simulink model "k1visbs"  (Simulink 8.5)
settings: Solver=ode45  StartTime=0.0  StopTime=10.0  RelTol=1e-3
undefined symbols (not defined in the file): AC, FOUROSEM_OPLEV_DAMP_MASTER, SIXOSEM_F_STAGE_MASTER, SIXOSEM_F_WD_AC_MASTER
libraries: cdsEpicsOut x82, cdsFilt x57, cdsTP x36, cdsFiltCtrl x16, VIS_LIB x14, cdsMuxMatrix x13, cdsEpicsIn x10, cdsEpicsBinIn x6, cdsRms x6, STATE_BIO_MASTER x4, lockin x4, cdsFunctionCall x4
(part 2 of 8)

== system k1visbs/BS/TEST ==
  In1 : Inport
  In4 : Inport  Port=2
  In7 : Inport  Port=3
  In10 : Inport  Port=4
  CH1 : cdsFiltCtrl/IIR FM with control  Tag=cdsFiltCtrl  Description=|
      | cdsFiltCntrl is the standard IIR filter module (exactly the same as cdsFilt) but with added control data output 'Ctrl'. Filter module digital signal output appears on the first output, which is called 'Val'. 'Ctrl' output has a bit pattern encoding the state of filter's on/off switches (FM1 through FM10). The bit values are:
      |                                                                                                                                                                                                                                                                                                                                       
      | module 	hex	dec                                                                                                                                                                                                                                                                                                                       
      | -----------------------                                                                                                                                                                                                                                                                                                               
      | FM1	0x20                    32                                                                                                                                                                                                                                                                                                        
      | FM2	0x80                     128                                                                                                                                                                                                                                                                                                      
      | FM3	0x200                   512                                                                                                                                                                                                                                                                                                       
      | FM4	0x800                   2048                                                                                                                                                                                                                                                                                                      
      | FM5	0x2000                 8192                                                                                                                                                                                                                                                                                                       
      | FM6	0x8000                 32768                                                                                                                                                                                                                                                                                                      
      | FM7	0x20000                131072                                                                                                                                                                                                                                                                                                     
      | FM8	0x80000                 524288                                                                                                                                                                                                                                                                                                    
      | FM9	0x200000               2097152                                                                                                                                                                                                                                                                                                    
      | FM10	0x800000               8388608                                                                                                                                                                                                                                                                                                   
      |                                                                                                                                                                                                                                                                                                                                       
      | This bit data can be used to drive some other switches or it can be output using a binary I/O module.
      settings: AttributesFormatString=%<Tag>
  CH2 : cdsFiltCtrl/IIR FM with control  Tag=cdsFiltCtrl  Description=|
      | cdsFiltCntrl is the standard IIR filter module (exactly the same as cdsFilt) but with added control data output 'Ctrl'. Filter module digital signal output appears on the first output, which is called 'Val'. 'Ctrl' output has a bit pattern encoding the state of filter's on/off switches (FM1 through FM10). The bit values are:
      |                                                                                                                                                                                                                                                                                                                                       
      | module 	hex	dec                                                                                                                                                                                                                                                                                                                       
      | -----------------------                                                                                                                                                                                                                                                                                                               
      | FM1	0x20                    32                                                                                                                                                                                                                                                                                                        
      | FM2	0x80                     128                                                                                                                                                                                                                                                                                                      
      | FM3	0x200                   512                                                                                                                                                                                                                                                                                                       
      | FM4	0x800                   2048                                                                                                                                                                                                                                                                                                      
      | FM5	0x2000                 8192                                                                                                                                                                                                                                                                                                       
      | FM6	0x8000                 32768                                                                                                                                                                                                                                                                                                      
      | FM7	0x20000                131072                                                                                                                                                                                                                                                                                                     
      | FM8	0x80000                 524288                                                                                                                                                                                                                                                                                                    
      | FM9	0x200000               2097152                                                                                                                                                                                                                                                                                                    
      | FM10	0x800000               8388608                                                                                                                                                                                                                                                                                                   
      |                                                                                                                                                                                                                                                                                                                                       
      | This bit data can be used to drive some other switches or it can be output using a binary I/O module.
      settings: AttributesFormatString=%<Tag>
  CH3 : cdsFiltCtrl/IIR FM with control  Tag=cdsFiltCtrl  Description=|
      | cdsFiltCntrl is the standard IIR filter module (exactly the same as cdsFilt) but with added control data output 'Ctrl'. Filter module digital signal output appears on the first output, which is called 'Val'. 'Ctrl' output has a bit pattern encoding the state of filter's on/off switches (FM1 through FM10). The bit values are:
      |                                                                                                                                                                                                                                                                                                                                       
      | module 	hex	dec                                                                                                                                                                                                                                                                                                                       
      | -----------------------                                                                                                                                                                                                                                                                                                               
      | FM1	0x20                    32                                                                                                                                                                                                                                                                                                        
      | FM2	0x80                     128                                                                                                                                                                                                                                                                                                      
      | FM3	0x200                   512                                                                                                                                                                                                                                                                                                       
      | FM4	0x800                   2048                                                                                                                                                                                                                                                                                                      
      | FM5	0x2000                 8192                                                                                                                                                                                                                                                                                                       
      | FM6	0x8000                 32768                                                                                                                                                                                                                                                                                                      
      | FM7	0x20000                131072                                                                                                                                                                                                                                                                                                     
      | FM8	0x80000                 524288                                                                                                                                                                                                                                                                                                    
      | FM9	0x200000               2097152                                                                                                                                                                                                                                                                                                    
      | FM10	0x800000               8388608                                                                                                                                                                                                                                                                                                   
      |                                                                                                                                                                                                                                                                                                                                       
      | This bit data can be used to drive some other switches or it can be output using a binary I/O module.
      settings: AttributesFormatString=%<Tag>
  CH4 : cdsFiltCtrl/IIR FM with control  Tag=cdsFiltCtrl  Description=|
      | cdsFiltCntrl is the standard IIR filter module (exactly the same as cdsFilt) but with added control data output 'Ctrl'. Filter module digital signal output appears on the first output, which is called 'Val'. 'Ctrl' output has a bit pattern encoding the state of filter's on/off switches (FM1 through FM10). The bit values are:
      |                                                                                                                                                                                                                                                                                                                                       
      | module 	hex	dec                                                                                                                                                                                                                                                                                                                       
      | -----------------------                                                                                                                                                                                                                                                                                                               
      | FM1	0x20                    32                                                                                                                                                                                                                                                                                                        
      | FM2	0x80                     128                                                                                                                                                                                                                                                                                                      
      | FM3	0x200                   512                                                                                                                                                                                                                                                                                                       
      | FM4	0x800                   2048                                                                                                                                                                                                                                                                                                      
      | FM5	0x2000                 8192                                                                                                                                                                                                                                                                                                       
      | FM6	0x8000                 32768                                                                                                                                                                                                                                                                                                      
      | FM7	0x20000                131072                                                                                                                                                                                                                                                                                                     
      | FM8	0x80000                 524288                                                                                                                                                                                                                                                                                                    
      | FM9	0x200000               2097152                                                                                                                                                                                                                                                                                                    
      | FM10	0x800000               8388608                                                                                                                                                                                                                                                                                                   
      |                                                                                                                                                                                                                                                                                                                                       
      | This bit data can be used to drive some other switches or it can be output using a binary I/O module.
      settings: AttributesFormatString=%<Tag>
  Ground{1..6,19,22} (8 alike) : Ground
  Terminator{1..5,16..18} (8 alike) : Terminator
  wires:
  CH4/2 -> Terminator1/1
  Ground5/1 -> CH4/3
  Ground6/1 -> CH4/2
  Ground3/1 -> CH3/3
  Ground4/1 -> CH3/2
  Ground1/1 -> CH2/3
  Ground2/1 -> CH2/2
  CH3/2 -> Terminator18/1
  CH2/2 -> Terminator17/1
  CH1/2 -> Terminator16/1
  Ground19/1 -> CH1/3
  Ground22/1 -> CH1/2
  In10/1 -> CH4/1
  In7/1 -> CH3/1
  In1/1 -> CH1/1
  CH2/1 -> Terminator4/1
  In4/1 -> CH2/1
  CH4/1 -> Terminator2/1
  CH3/1 -> Terminator3/1
  CH1/1 -> Terminator5/1

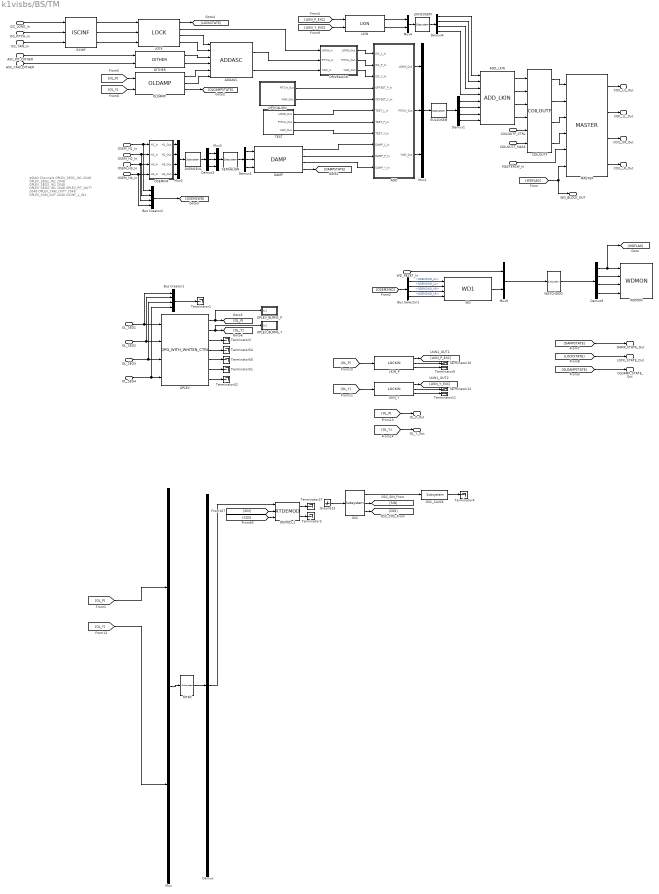
== system k1visbs/BS/TM ==
  note: #DAQ Channels
      | OPLEV_SEG1_IN1 2048
      | OPLEV_SEG2_IN1 2048
      | OPLEV_SEG3_IN1 2048
      | OPLEV_SEG4_IN1 2048
      | OPLEV_PIT_OUT* 2048
      | OPLEV_YAW_OUT* 2048
      | OPLEV_SUM_OUT 2048
      | ISCINF_L_IN1 2048
  OSEM_H1_In : Inport
  OSEM_H2_In : Inport  Port=2
  OSEM_H3_In : Inport  Port=3
  OSEM_H4_In : Inport  Port=4
  ISC_LONG_In : Inport  Port=5
  ISC_PITCH_In : Inport  Port=6
  ISC_YAW_In : Inport  Port=7
  COILOUTF_CTRL : Inport  Port=8
  COILOUTF_MASK : Inport  Port=9
  OL_SEG1 : Inport  Port=10
  OL_SEG2 : Inport  Port=11
  OL_SEG3 : Inport  Port=12
  OL_SEG4 : Inport  Port=13
  MASTERSW_In : Inport  Port=14
  WD_RESET_In : Inport  Port=15
  ASC_PIT_DITHER : Inport  Port=16
  ASC_YAW_DITHER : Inport  Port=17
  ADD : Subsystem
  ADDASC : VIS_LIB/ADDASC
  ADD_LKIN : VIS_LIB/ADD_LKIN
  Bus Creator1 : BusCreator  Inputs='OSEM2WD_UL','OSEM2WD_LL','OSEM2WD_UR','OSEM2WD_LR'
  Bus Creator2 : BusCreator  Inputs='OSEM2WD_UL','OSEM2WD_LL','OSEM2WD_UR','OSEM2WD_LR'
  Bus Selector1 : BusSelector  OutputSignals=OSEM2WD_UL,OSEM2WD_LL,OSEM2WD_UR,OSEM2WD_LR
  COILOUTF : FOUROSEM_COILOUTF_MASTER/COILOUTF
  DAMP : VIS_LIB/DAMP
  DEMOD_1 : rtdemod/RTDEMOD  Tag=top_names
  DITHER : VIS_LIB/DITHER
  DRIVEALIGN : Subsystem
  Demux : Demux  Outputs=1
  Demux1 : Demux
  Demux2 : Demux  Outputs=3
  Demux3 : Demux  Outputs=3
  Demux4 : Demux
  Demux9 : Demux
  EUL2OSEM : cdsMuxMatrix/Subsystem  Tag=cdsMuxMatrix  Description=Any size matrix. Inputs and outputs must be connected using Mux and Demux parts.
      settings: AttributesFormatString=%<Tag>
  Ground23 : Ground
  ISCINF : VIS_LIB/ISCINF
  LKIN : VIS_LIB/LKIN
  LKIN2OSEM : cdsMuxMatrix/Subsystem  Tag=cdsMuxMatrix  Description=Any size matrix. Inputs and outputs must be connected using Mux and Demux parts.
      settings: AttributesFormatString=%<Tag>
  LKIN_P : lockin/LOCKIN  Description=ADL=LOCKIN.adl
      settings: AttributesFormatString=%<Tag>
  LKIN_Y : lockin/LOCKIN  Description=ADL=LOCKIN.adl
      settings: AttributesFormatString=%<Tag>
  LOCK : VIS_LIB/LOCK
  MASTER : VIS_LIB/MASTER
  MTRX : cdsMuxMatrix/Subsystem  Tag=cdsMuxMatrix  Description=Any size matrix. Inputs and outputs must be connected using Mux and Demux parts.
      settings: AttributesFormatString=%<Tag>
  Mux : Mux  Inputs=2
  Mux1 : Mux  Inputs=3
  Mux2 : Mux
  Mux3 : Mux  Inputs=3
  Mux4 : Mux  Inputs=2
  Mux9 : Mux  Inputs=2
  OLDAMP : VIS_LIB/OLDAMP
  OPLEV : QPD/QPD_WITH_WHITEN_CTRL
  OPLEV_BLRMS_P : Subsystem
  OPLEV_BLRMS_Y : Subsystem
  OPTICALIGN : Subsystem
  OSC : cdsOsc/Subsystem  Tag=cdsOsc  Description=Oscillator
      settings: AttributesFormatString=%<Tag>
  OSC_CLOCK : cdsEpicsOut/Subsystem  Tag=cdsEpicsOutput  Description=|
      | Purpose:                                          
      | Output a FE signal to an EPICS channel.           
      |                                                   
      | Operation:                                        
      | Takes input value and passes it to EPICS record.  
      |                                                   
      | Usage:                                            
      | Name the part with the desired EPICS rrecord name.
      settings: AttributesFormatString=%<Tag>
  OSEM2EUL : cdsMuxMatrix/Subsystem  Tag=cdsMuxMatrix  Description=Any size matrix. Inputs and outputs must be connected using Mux and Demux parts.
      settings: AttributesFormatString=%<Tag>
  OSEMINF : Subsystem
  SENSALIGN : cdsMuxMatrix/Subsystem  Tag=cdsMuxMatrix  Description=Any size matrix. Inputs and outputs must be connected using Mux and Demux parts.
      settings: AttributesFormatString=%<Tag>
  TEST : Subsystem
  Terminator{1..4,9..12,27,50..52,54} (13 alike) : Terminator
  WATCHDOG : cdsFunctionCall/Subsystem  Tag=cdsFunctionCall  Description=inline OSEMWATCHDOG /opt/rtcds/userapps/release/vis/common/src/WATCHDOG.c
      settings: AttributesFormatString=%<Tag>\n%<Description>
  WD : VIS_LIB/WD1
  WDMON : VIS_LIB/WDMON
  COIL_UL_Out : Outport
  COIL_LL_Out : Outport  Port=2
  COIL_UR_Out : Outport  Port=3
  COIL_LR_Out : Outport  Port=4
  WD_BLOCK_OUT : Outport  Port=5
  DAMP_STATE_Out : Outport  Port=6
  LOCK_STATE_Out : Outport  Port=7
  OLDAMP_STATE_Out : Outport  Port=8
  OL_P_Out : Outport  Port=9
  OL_Y_Out : Outport  Port=10
  wires:
  [OL_Y] -> OL_Y_Out/1
  [OL_P] -> OL_P_Out/1
  [OL_Y] -> Mux/2
  [OL_P] -> Mux/1
  OSC/3 -> [COS]
  OSC/2 -> [SIN]
  OSC_CLOCK/1 -> Terminator4/1
  OSC/1 -> OSC_CLOCK/1
  Ground23/1 -> OSC/1
  DEMOD_1/2 -> Terminator3/1
  DEMOD_1/1 -> Terminator27/1
  [COS] -> DEMOD_1/3
  [SIN] -> DEMOD_1/2
  Demux/1 -> DEMOD_1/1
  MTRX/1 -> Demux/1
  Mux/1 -> MTRX/1
  ISCINF/3 -> LOCK/3
  ISCINF/2 -> LOCK/2
  ISCINF/1 -> LOCK/1
  ISC_PITCH_In/1 -> ISCINF/2
  ISC_LONG_In/1 -> ISCINF/1
  ISC_YAW_In/1 -> ISCINF/3
  WD/1 -> Mux9/2
  [LKIN_Y_EXC] -> LKIN/2
  [LKIN_P_EXC] -> LKIN/1
  LKIN_Y/3 -> Terminator11/1
  LKIN_Y/2 -> Terminator12/1
  [OL_Y] -> LKIN_Y/1
  LKIN_Y/1 -> [LKIN_Y_EXC]
  LKIN_P/1 -> [LKIN_P_EXC]
  LKIN_P/3 -> Terminator9/1
  LKIN_P/2 -> Terminator10/1
  [OL_P] -> LKIN_P/1
  DAMP/3 -> ADD/11(DAMP_Y_In)
  DAMP/2 -> ADD/10(DAMP_P_In)
  DAMP/1 -> ADD/9(DAMP_L_In)
  LOCK/1 -> [LOCKSTATE]
  DAMP/4 -> [DAMPSTATE]
  [OLDAMPSTATE] -> OLDAMP_STATE_Out/1
  [LOCKSTATE] -> LOCK_STATE_Out/1
  [DAMPSTATE] -> DAMP_STATE_Out/1
  MASTERSW_In/1 -> MASTER/5
  ADD_LKIN/4 -> COILOUTF/4
  ADD_LKIN/3 -> COILOUTF/3
  ADD_LKIN/2 -> COILOUTF/2
  ADD_LKIN/1 -> COILOUTF/1
  Demux1/4 -> ADD_LKIN/8
  Demux1/3 -> ADD_LKIN/7
  Demux1/2 -> ADD_LKIN/6
  Demux1/1 -> ADD_LKIN/5
  Demux4/4 -> ADD_LKIN/4
  Demux4/3 -> ADD_LKIN/3
  Demux4/2 -> ADD_LKIN/2
  LKIN/2 -> Mux4/2
  LKIN/1 -> Mux4/1
  Demux4/1 -> ADD_LKIN/1
  LKIN2OSEM/1 -> Demux4/1
  Mux4/1 -> LKIN2OSEM/1
  MASTER/4 -> COIL_LR_Out/1
  MASTER/3 -> COIL_UR_Out/1
  MASTER/2 -> COIL_LL_Out/1
  MASTER/1 -> COIL_UL_Out/1
  OPLEV/7 -> Terminator52/1
  OPLEV/6 -> Terminator51/1
  OPLEV/5 -> Terminator50/1
  OPLEV/4 -> Terminator54/1
  OLDAMP/3 -> [OLDAMPSTATE]
  OPLEV/3 -> Terminator2/1
  OPLEV/1 -> [OL_P], OPLEV_BLRMS_P/1(In1)
  OPLEV/2 -> [OL_Y], OPLEV_BLRMS_Y/1(In1)
  DRIVEALIGN/3(YAW_Out) -> ADD/3(ISC_Y_In)
  DRIVEALIGN/2(PITCH_Out) -> ADD/2(ISC_P_In)
  DRIVEALIGN/1(LONG_Out) -> ADD/1(ISC_L_In)
  ADDASC/2 -> DRIVEALIGN/3(YAW_In)
  ADDASC/1 -> DRIVEALIGN/2(PITCH_In)
  LOCK/2 -> DRIVEALIGN/1(LONG_In)
  ADD/1(LONG_Out) -> Mux1/1
  ADD/2(PITCH_Out) -> Mux1/2
  ADD/3(YAW_Out) -> Mux1/3
  OLDAMP/2 -> ADDASC/6
  OLDAMP/1 -> ADDASC/5
  DITHER/2 -> ADDASC/4
  DITHER/1 -> ADDASC/3
  LOCK/4 -> ADDASC/2
  [OL_Y] -> OLDAMP/2
  [OL_P] -> OLDAMP/1
  ASC_YAW_DITHER/1 -> DITHER/2
  ASC_PIT_DITHER/1 -> DITHER/1
  OL_SEG4/1 -> OPLEV/4, Bus Creator1/4
  OL_SEG3/1 -> Bus Creator1/3, OPLEV/3
  OL_SEG2/1 -> Bus Creator1/2, OPLEV/2
  OL_SEG1/1 -> OPLEV/1, Bus Creator1/1
  Bus Selector1/4 -> WD/4  "<OSEM2WD_LR>"
  Bus Selector1/3 -> WD/3  "<OSEM2WD_UR>"
  Bus Selector1/2 -> WD/2  "<OSEM2WD_LL>"
  Bus Selector1/1 -> WD/1  "<OSEM2WD_UL>"
  [OSEM2WD] -> Bus Selector1/1
  Demux2/3 -> DAMP/3
  Demux2/2 -> DAMP/2
  Demux2/1 -> DAMP/1
  OSEMINF/4(H4_Out) -> Mux2/4
  OSEMINF/3(H3_Out) -> Mux2/3
  OSEMINF/2(H2_Out) -> Mux2/2
  OSEMINF/1(H1_Out) -> Mux2/1
  OSEM_H4_In/1 -> Bus Creator2/4, OSEMINF/4(H4_In)
  OSEM_H3_In/1 -> Bus Creator2/3, OSEMINF/3(H3_In)
  OSEM_H2_In/1 -> Bus Creator2/2, OSEMINF/2(H2_In)
  OSEM_H1_In/1 -> Bus Creator2/1, OSEMINF/1(H1_In)
  Mux2/1 -> OSEM2EUL/1
  OSEM2EUL/1 -> Demux3/1
  Mux3/1 -> SENSALIGN/1
  SENSALIGN/1 -> Demux2/1
  Mux1/1 -> EUL2OSEM/1
  EUL2OSEM/1 -> Demux1/1
  Demux3/1 -> Mux3/1
  Demux3/2 -> Mux3/2
  Demux3/3 -> Mux3/3
  Demux9/1 -> [WDFLAG], WDMON/1
  Demux9/2 -> WDMON/2
  Demux9/3 -> WDMON/3
  Demux9/4 -> WDMON/4
  WATCHDOG/1 -> Demux9/1
  Mux9/1 -> WATCHDOG/1
  [WDFLAG] -> WD_BLOCK_OUT/1, MASTER/6
  COILOUTF/1 -> MASTER/1
  COILOUTF/2 -> MASTER/2
  COILOUTF/3 -> MASTER/3
  COILOUTF/4 -> MASTER/4
  WD_RESET_In/1 -> Mux9/1
  COILOUTF_MASK/1 -> COILOUTF/6
  COILOUTF_CTRL/1 -> COILOUTF/5
  TEST/1(LONG_Out) -> ADD/6(TEST_L_In)
  TEST/2(PITCH_Out) -> ADD/7(TEST_P_In)
  TEST/3(YAW_Out) -> ADD/8(TEST_Y_In)
  LOCK/3 -> ADDASC/1
  OPTICALIGN/1(PITCH_Out) -> ADD/4(OFFSET_P_In)
  OPTICALIGN/2(YAW_Out) -> ADD/5(OFFSET_Y_In)
  Bus Creator2/1 -> [OSEM2WD]
  Bus Creator1/1 -> Terminator1/1

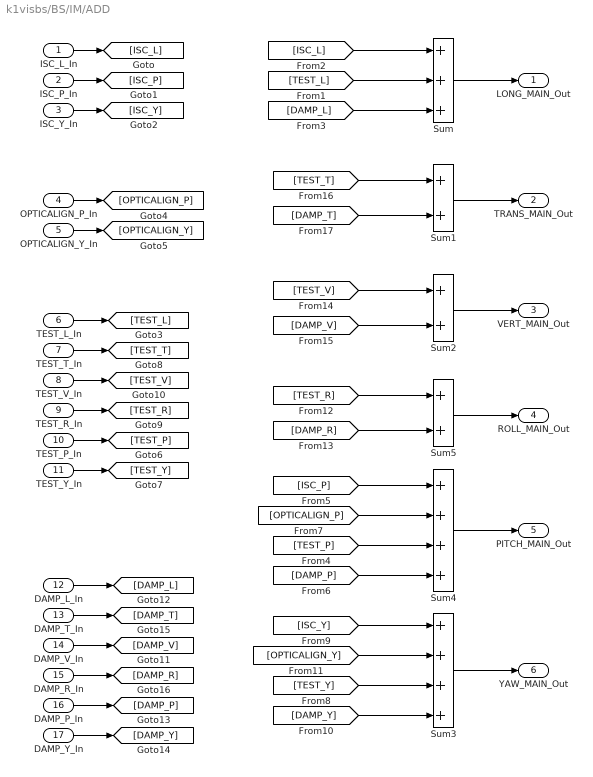
== system k1visbs/BS/IM/ADD ==
  ISC_L_In : Inport
  ISC_P_In : Inport  Port=2
  ISC_Y_In : Inport  Port=3
  OPTICALIGN_P_In : Inport  Port=4
  OPTICALIGN_Y_In : Inport  Port=5
  TEST_L_In : Inport  Port=6
  TEST_T_In : Inport  Port=7
  TEST_V_In : Inport  Port=8
  TEST_R_In : Inport  Port=9
  TEST_P_In : Inport  Port=10
  TEST_Y_In : Inport  Port=11
  DAMP_L_In : Inport  Port=12
  DAMP_T_In : Inport  Port=13
  DAMP_V_In : Inport  Port=14
  DAMP_R_In : Inport  Port=15
  DAMP_P_In : Inport  Port=16
  DAMP_Y_In : Inport  Port=17
  Sum : Sum  Inputs=+++
  Sum1 : Sum
  Sum2 : Sum
  Sum3 : Sum  Inputs=++++
  Sum4 : Sum  Inputs=++++
  Sum5 : Sum
  LONG_MAIN_Out : Outport
  TRANS_MAIN_Out : Outport  Port=2
  VERT_MAIN_Out : Outport  Port=3
  ROLL_MAIN_Out : Outport  Port=4
  PITCH_MAIN_Out : Outport  Port=5
  YAW_MAIN_Out : Outport  Port=6
  wires:
  [DAMP_V] -> Sum2/2
  [TEST_V] -> Sum2/1
  [DAMP_T] -> Sum1/2
  [TEST_T] -> Sum1/1
  [DAMP_R] -> Sum5/2
  [TEST_R] -> Sum5/1
  [DAMP_Y] -> Sum3/4
  [TEST_Y] -> Sum3/3
  [OPTICALIGN_Y] -> Sum3/2
  [ISC_Y] -> Sum3/1
  [DAMP_P] -> Sum4/4
  [TEST_P] -> Sum4/3
  [OPTICALIGN_P] -> Sum4/2
  [ISC_P] -> Sum4/1
  DAMP_Y_In/1 -> [DAMP_Y]
  DAMP_P_In/1 -> [DAMP_P]
  DAMP_R_In/1 -> [DAMP_R]
  DAMP_V_In/1 -> [DAMP_V]
  DAMP_T_In/1 -> [DAMP_T]
  DAMP_L_In/1 -> [DAMP_L]
  TEST_Y_In/1 -> [TEST_Y]
  TEST_P_In/1 -> [TEST_P]
  TEST_R_In/1 -> [TEST_R]
  TEST_V_In/1 -> [TEST_V]
  TEST_T_In/1 -> [TEST_T]
  TEST_L_In/1 -> [TEST_L]
  ISC_Y_In/1 -> [ISC_Y]
  ISC_P_In/1 -> [ISC_P]
  ISC_L_In/1 -> [ISC_L]
  OPTICALIGN_Y_In/1 -> [OPTICALIGN_Y]
  OPTICALIGN_P_In/1 -> [OPTICALIGN_P]
  Sum1/1 -> TRANS_MAIN_Out/1
  Sum2/1 -> VERT_MAIN_Out/1
  Sum5/1 -> ROLL_MAIN_Out/1
  [DAMP_L] -> Sum/3
  [TEST_L] -> Sum/2
  [ISC_L] -> Sum/1
  Sum/1 -> LONG_MAIN_Out/1
  Sum3/1 -> YAW_MAIN_Out/1
  Sum4/1 -> PITCH_MAIN_Out/1

== system k1visbs/BS/IM/ADD_LKIN ==
  LKN_V1_In : Inport
  LKN_V2_In : Inport  Port=2
  LKIN_V3_In : Inport  Port=3
  LKIN_H1_In : Inport  Port=4
  LKIN_H2_In : Inport  Port=5
  LKIN_H3_In : Inport  Port=6
  OSEM_V1_In : Inport  Port=7
  OSEM_V2_In : Inport  Port=8
  OSEM_V3_In : Inport  Port=9
  OSEM_H1_In : Inport  Port=10
  OSEM_H2_In : Inport  Port=11
  OSEM_H3_In : Inport  Port=12
  Sum{,1..5} (6 alike) : Sum
  V1_Out : Outport
  V2_Out : Outport  Port=2
  V3_Out : Outport  Port=3
  H1_Out : Outport  Port=4
  H2_Out : Outport  Port=5
  H3_Out : Outport  Port=6
  wires:
  LKIN_H3_In/1 -> Sum2/1
  LKIN_H2_In/1 -> Sum5/1
  Sum5/1 -> H2_Out/1
  OSEM_H2_In/1 -> Sum5/2
  Sum2/1 -> H3_Out/1
  OSEM_H3_In/1 -> Sum2/2
  LKIN_H1_In/1 -> Sum1/1
  LKIN_V3_In/1 -> Sum3/1
  LKN_V2_In/1 -> Sum4/1
  Sum/1 -> V1_Out/1
  LKN_V1_In/1 -> Sum/1
  OSEM_V1_In/1 -> Sum/2
  Sum3/1 -> V3_Out/1
  Sum4/1 -> V2_Out/1
  OSEM_V3_In/1 -> Sum3/2
  OSEM_V2_In/1 -> Sum4/2
  Sum1/1 -> H1_Out/1
  OSEM_H1_In/1 -> Sum1/2
